simulink model "symulacja"  (R2017b)
settings: Solver=FixedStepAuto  StartTime=0.0  StopTime=10.0  FixedStep=Tp  RelTol=1e-3  EnableMultiTasking=on
values from neighbouring files (symbols this model uses):
  FV = 1    [projekt2.m]
  K = 1.4    [projekt2.m]
  T1 = 1/14    (= 0.0714285714286)    [projekt2.m]
  T2 = 100    [projekt2.m]
  T3 = 10    [projekt2.m]
  T4 = 1    [projekt2.m]
settings Model: Creator=Alicja  LastModifiedBy=Alicja
settings DataIOCC: SaveFormat=Array  OutputSaveName=u,y

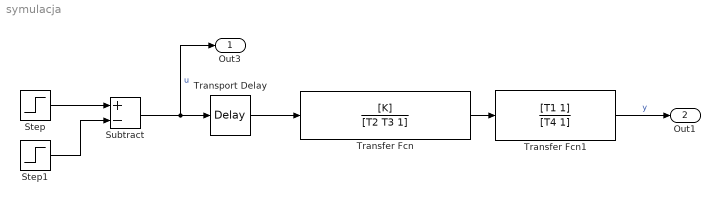
== system symulacja ==
  Step : Step  Time=10  SampleTime=0
  Step1 : Step  Time=11  After=FV  SampleTime=0
  Subtract : Sum  Inputs=+-
  Transfer Fcn : TransferFcn  Numerator=[K]  Denominator=[T2 T3 1]
  Transfer Fcn1 : TransferFcn  Numerator=[T1 1]  Denominator=[T4 1]
  Transport Delay : TransportDelay  DelayTime=20
  Out3 : Outport
  Out1 : Outport  Port=2
  wires:
  Transport Delay/1 -> Transfer Fcn/1
  Transfer Fcn1/1 -> Out1/1  "y"
  Subtract/1 -> Out3/1, Transport Delay/1  "u"
  Step/1 -> Subtract/1
  Step1/1 -> Subtract/2
  Transfer Fcn/1 -> Transfer Fcn1/1
